simulink model "MSE483Project_StateSpaceForm"  (R2020b)
settings: Solver=VariableStepAuto  StartTime=0.0  StopTime=8  RelTol=1e-3
InitFcn:
  | A=[0,  0,           1,          0;
  |     0,  0,           0,          1;
  |     0, -409.7184,  -104.6299,   104.6299;
  |     0,  268.6273,    54.5833,   -54.5833]
  | B = [0;0;101.6952;-53.0523]
  | C=[1,0,0,0;0,1,0,0;0,0,1,0;0,0,0,1]
  | D=[0]
  | x0=[0;90*pi/180;0;0]
  | K = [-120.259117270779, -408.292835208155, -22.2596920604937, -43.0045547926153]
  | Ob= [ 400.0000   ,      0   , 1.0000  ,       0;
  |          0 , 400.0000   ,      0  ,  1.0000;
  |          0, -409.718, 295.3701 , 104.6299;
  |          0,  268.6273 ,  54.5833 , 345.4167]
settings Model: Creator=samuel  LastModifiedBy=samuel

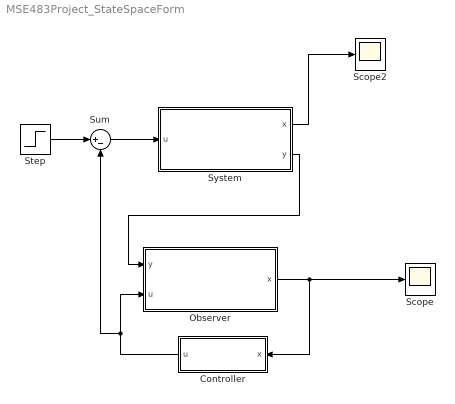
== system MSE483Project_StateSpaceForm ==
  Controller : Subsystem
  Observer : Subsystem
  Scope : Scope
  Scope2 : Scope
  Step : Step  Before=1  After=0  SampleTime=0
  Sum : Sum  Inputs=|+-
  System : Subsystem
  wires:
  Step/1 -> Sum/1
  Sum/1 -> System/1(u)
  System/2(y) -> Observer/1(y)
  Controller/1(u) -> Observer/2(u), Sum/2
  System/1(x) -> Scope2/1
  Observer/1(x) -> Controller/1(x), Scope/1

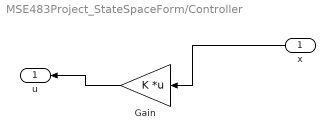
== system MSE483Project_StateSpaceForm/Controller ==
  x : Inport
  Gain : Gain  Gain=K  Multiplication=Matrix(K*u)
  u : Outport
  wires:
  Gain/1 -> u/1
  x/1 -> Gain/1

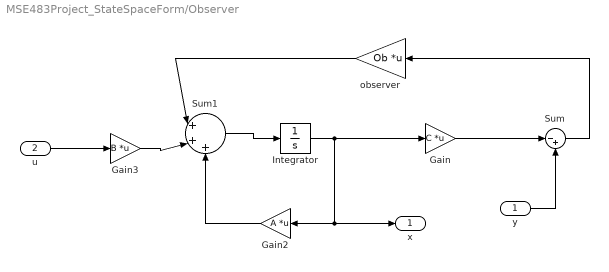
== system MSE483Project_StateSpaceForm/Observer ==
  y : Inport
  u : Inport  Port=2
  Gain : Gain  Gain=C  Multiplication=Matrix(K*u)
  Gain2 : Gain  Gain=A  Multiplication=Matrix(K*u)
  Gain3 : Gain  Gain=B  Multiplication=Matrix(K*u)
  Integrator : Integrator  InitialCondition=x0
  Sum : Sum  Inputs=|-+
  Sum1 : Sum  Inputs=|+++
  observer : Gain  Gain=Ob  Multiplication=Matrix(K*u)
  x : Outport
  wires:
  u/1 -> Gain3/1
  Gain/1 -> Sum/1
  Sum1/1 -> Integrator/1
  Integrator/1 -> Gain2/1, x/1, Gain/1
  y/1 -> Sum/2
  Sum/1 -> observer/1
  observer/1 -> Sum1/1
  Gain3/1 -> Sum1/2
  Gain2/1 -> Sum1/3

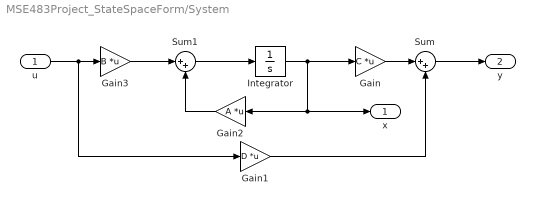
== system MSE483Project_StateSpaceForm/System ==
  u : Inport
  Gain : Gain  Gain=C  Multiplication=Matrix(K*u)
  Gain1 : Gain  Gain=D  Multiplication=Matrix(K*u)
  Gain2 : Gain  Gain=A  Multiplication=Matrix(K*u)
  Gain3 : Gain  Gain=B  Multiplication=Matrix(K*u)
  Integrator : Integrator  InitialCondition=x0
  Sum : Sum  Inputs=|++
  Sum1 : Sum  Inputs=|++
  x : Outport
  y : Outport  Port=2
  wires:
  Integrator/1 -> Gain2/1, x/1, Gain/1
  u/1 -> Gain1/1, Gain3/1
  Gain/1 -> Sum/1
  Sum1/1 -> Integrator/1
  Gain2/1 -> Sum1/2
  Gain3/1 -> Sum1/1
  Sum/1 -> y/1
  Gain1/1 -> Sum/2
